simulink model "model"  (R2024a)
settings: Solver=VariableStepAuto  StartTime=0.0  StopTime=85  RelTol=1e-3
values from neighbouring files (symbols this model uses):
  b = 0.5*CdA*rho    (= 0.3316545)    [init.m]    (also in stateFcnTaycan.m)
  F_max = [22000 1710]    [init.m]    (also in stateFcnTaycan.m = interp1(v_to_F_max_lu, F_max_lu, v, 'linear'))
  F_min = -20000    [init.m]    (also in stateFcnTaycan.m)
  m = 2140    [init.m]    (also in stateFcnTaycan.m)
  Ts = 1    [init.m]
  v_to_F_max = [0 72]    [init.m]
libraries: simulink x2, mpclib x1
settings Model: Creator=berto  LastModifiedBy=berto

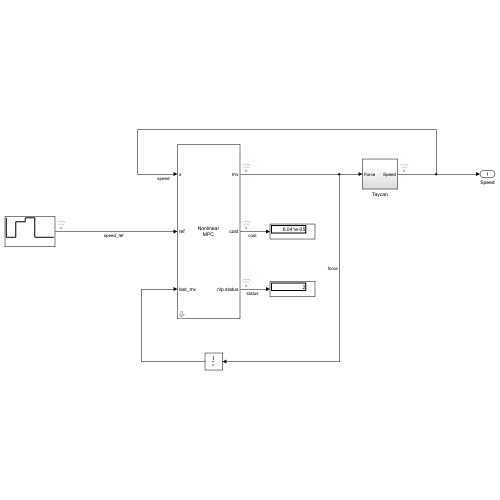
[thumbnail: Simulink's stored preview of the top-level diagram]
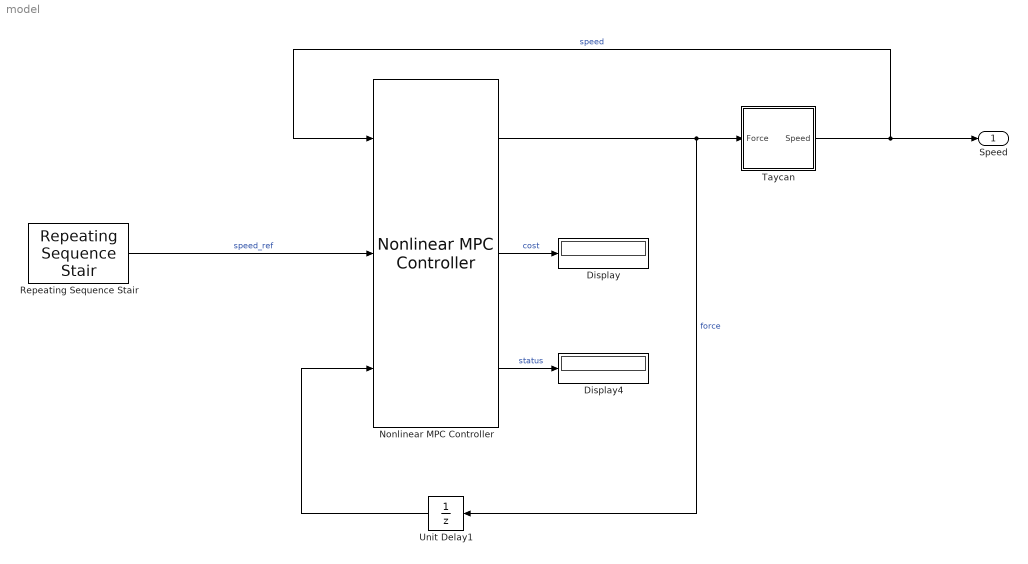
== system model ==
  Display : Display
  Display4 : Display
  Nonlinear MPC Controller : mpclib/Nonlinear MPC Controller  nlmpcobj=nlobj  UseObjectTs=on  UseMEX=off  md_enabled=off  mvtarget_enabled=off  param_enabled=off  cost_enabled=on  mvseq_enabled=off  stateseq_enabled=off  ovseq_enabled=off  slack_enabled=off  status_enabled=on  ov_min=off  ov_max=off  mv_min=off  mv_max=off  mvrate_min=off  mvrate_max=off  state_min=off  state_max=off  ov_weight=off  mv_weight=off  mvrate_weight=off  ecr_weight=off  nlp_initialize=off
  Repeating Sequence Stair : simulink/Sources/Repeating Sequence Stair  OutValues=[10 50 60 10 10].'  tsamp=20  OutMin=[]  OutMax=[]  OutDataTypeStr=double  OutputDataTypeScalingMode=double  OutDataType=fixdt(0,8)  ConRadixGroup=Best Precision: Vector-wise  OutScaling=2^-12
  Taycan : Subsystem
  Unit Delay1 : UnitDelay  SampleTime=Ts  HasFrameUpgradeWarning=on
  Speed : Outport
  wires:
  Taycan/1(Speed) -> Nonlinear MPC Controller/1, Speed/1  "speed"
  Nonlinear MPC Controller/1 -> Taycan/1(Force), Unit Delay1/1  "force"
  Repeating Sequence Stair/1 -> Nonlinear MPC Controller/2  "speed_ref"
  Unit Delay1/1 -> Nonlinear MPC Controller/3
  Nonlinear MPC Controller/2 -> Display/1  "cost"
  Nonlinear MPC Controller/3 -> Display4/1  "status"

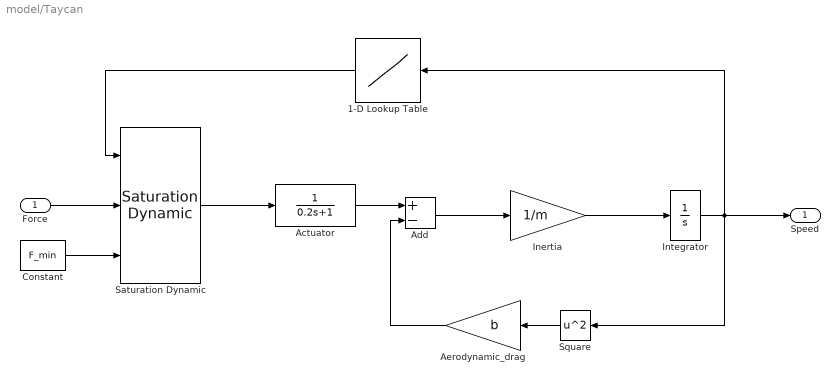
== system model/Taycan ==
  Force : Inport
  1-D Lookup Table : Lookup_n-D  NumberOfTableDimensions=1  BreakpointsForDimension1=v_to_F_max  Table=F_max  ExtrapMethod=Clip  InternalRulePriority=Speed  RndMeth=Simplest
  Actuator : TransferFcn  Denominator=[0.2 1]
  Add : Sum  Inputs=+-
  Aerodynamic_drag : Gain  Gain=b
  Constant : Constant  Value=F_min
  Inertia : Gain  Gain=1/m
  Integrator : Integrator
  Saturation Dynamic : simulink/Discontinuities/Saturation Dynamic  OutMin=[]  OutMax=[]  OutDataTypeStr=Inherit: Same as second input  OutDataType=fixdt(1, 16)  OutScaling=2^-10  DoSatur=off
  Square : Math  Operator=square
  Speed : Outport
  wires:
  Force/1 -> Saturation Dynamic/2
  Actuator/1 -> Add/1
  Integrator/1 -> Speed/1, 1-D Lookup Table/1, Square/1
  Constant/1 -> Saturation Dynamic/3
  Saturation Dynamic/1 -> Actuator/1
  1-D Lookup Table/1 -> Saturation Dynamic/1
  Aerodynamic_drag/1 -> Add/2
  Add/1 -> Inertia/1
  Inertia/1 -> Integrator/1
  Square/1 -> Aerodynamic_drag/1
